simulink model "Lab01R1Sim"  (Simulink 7.1)
settings: Solver=ode45  StartTime=0.0  StopTime=10  RelTol=1e-3
settings Model: Creator=CARLOS BRUNO  LastModifiedBy=CARLOS BRUNO
settings OptimizationCC: InlineInvariantSignals=on
settings DebuggingCC: SaveWithParameterizedLinksMsg=none  SignalResolutionControl=TryResolveAllWithWarning  MultiTaskDSMMsg=warning  MultiTaskCondExecSysMsg=none  StrictBusMsg=None
settings RTWCC: IncludeERTFirstTime=on
settings GRTTargetCC: TargetFcnLib=ansi_tfl_tmw.mat

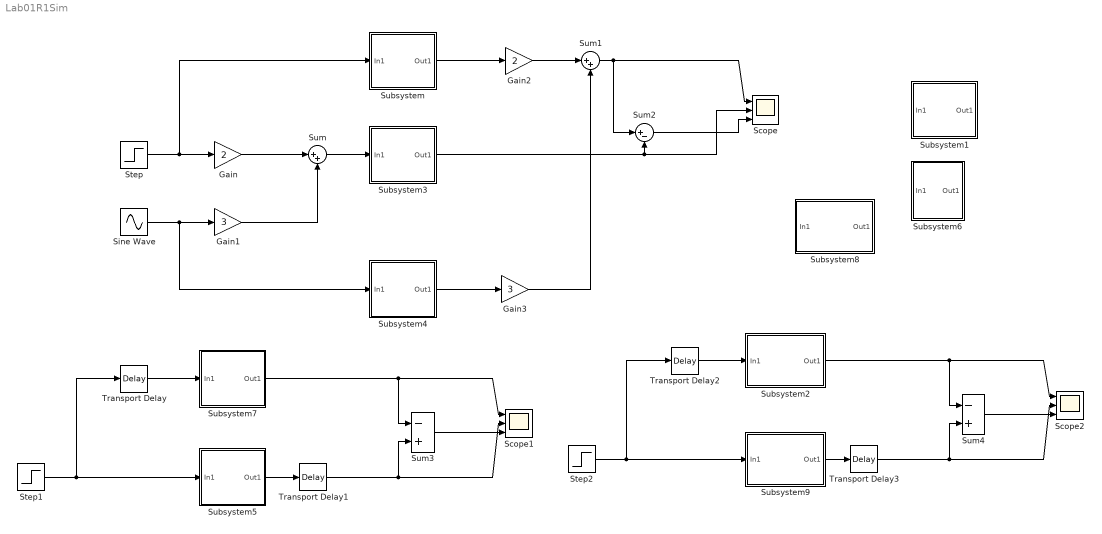
== system Lab01R1Sim ==
  Gain : Gain  Gain=2  ParameterDataType=sfix(16)  ParameterScaling=2^0  OutDataType=sfix(16)  OutScaling=2^0
  Gain1 : Gain  Gain=3  ParameterDataType=sfix(16)  ParameterScaling=2^0  OutDataType=sfix(16)  OutScaling=2^0
  Gain2 : Gain  Gain=2  ParameterDataType=sfix(16)  ParameterScaling=2^0  OutDataType=sfix(16)  OutScaling=2^0
  Gain3 : Gain  Gain=3  ParameterDataType=sfix(16)  ParameterScaling=2^0  OutDataType=sfix(16)  OutScaling=2^0
  Scope : Scope  NumInputPorts=3
      settings: TimeRange=10  YMin=-5~-5~-2e-015  YMax=20~20~4e-015
  Scope1 : Scope  NumInputPorts=3
      settings: TimeRange=10  YMin=-5~-5~-2e-015  YMax=20~20~4e-015
  Scope2 : Scope  NumInputPorts=3
      settings: TimeRange=10  YMin=-5~-5~-2e-015  YMax=20~20~4e-015  SaveName=ScopeData2
  Sine Wave : Sin  SampleTime=0
  Step : Step  Time=0  SampleTime=0
  Step1 : Step  Time=0  SampleTime=0
  Step2 : Step  Time=0  SampleTime=0
  Subsystem : Subsystem
      mask Display: disp('Planta P1')
  Subsystem1 : Subsystem
      mask Display: disp('Planta P2')
  Subsystem2 : Subsystem
      mask Display: disp('Planta P4')
  Subsystem3 : Subsystem
      mask Display: disp('Planta P1')
  Subsystem4 : Subsystem
      mask Display: disp('Planta P1')
  Subsystem5 : Subsystem
      mask Display: disp('Planta P1')
  Subsystem6 : Subsystem
      mask Display: disp('Planta P3')
  Subsystem7 : Subsystem
      mask Display: disp('Planta P1')
  Subsystem8 : Subsystem
      mask Display: disp('Planta P4')
  Subsystem9 : Subsystem
      mask Display: disp('Planta P4')
  Sum : Sum  Inputs=|++  OutDataType=sfix(16)  OutScaling=2^0
  Sum1 : Sum  Inputs=|++  OutDataType=sfix(16)  OutScaling=2^0
  Sum2 : Sum  Inputs=|+-  OutDataType=sfix(16)  OutScaling=2^0
  Sum3 : Sum  Inputs=|-+  OutDataType=sfix(16)  OutScaling=2^0
  Sum4 : Sum  Inputs=|-+  OutDataType=sfix(16)  OutScaling=2^0
  Transport Delay{,1..3} (4 alike) : TransportDelay
  wires:
  Step/1 -> Gain/1, Subsystem/1(In1)
  Sine Wave/1 -> Gain1/1, Subsystem4/1(In1)
  Gain/1 -> Sum/1
  Sum/1 -> Subsystem3/1(In1)
  Gain1/1 -> Sum/2
  Subsystem4/1(Out1) -> Gain3/1
  Subsystem/1(Out1) -> Gain2/1
  Gain2/1 -> Sum1/1
  Gain3/1 -> Sum1/2
  Subsystem3/1(Out1) -> Sum2/2, Scope/2
  Sum1/1 -> Scope/1, Sum2/1
  Sum2/1 -> Scope/3
  Step1/1 -> Transport Delay/1, Subsystem5/1(In1)
  Transport Delay/1 -> Subsystem7/1(In1)
  Subsystem5/1(Out1) -> Transport Delay1/1
  Subsystem7/1(Out1) -> Sum3/1, Scope1/1
  Transport Delay1/1 -> Sum3/2, Scope1/2
  Sum3/1 -> Scope1/3
  Step2/1 -> Transport Delay2/1, Subsystem9/1(In1)
  Transport Delay2/1 -> Subsystem2/1(In1)
  Subsystem2/1(Out1) -> Sum4/1, Scope2/1
  Transport Delay3/1 -> Sum4/2, Scope2/2
  Sum4/1 -> Scope2/3
  Subsystem9/1(Out1) -> Transport Delay3/1

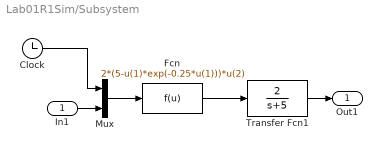
== system Lab01R1Sim/Subsystem ==
  In1 : Inport  OutDataType=sfix(16)  OutScaling=2^0
  Clock : Clock
      settings: Decimation=10
  Fcn : Fcn  Expr=2*(5-u(1)*exp(-0.25*u(1)))*u(2)
  Mux : Mux  Inputs=2
  Transfer Fcn1 : TransferFcn  Numerator=[2]  Denominator=[1 5]
  Out1 : Outport  OutDataType=sfix(16)  OutScaling=2^0
  wires:
  Clock/1 -> Mux/1
  Mux/1 -> Fcn/1
  Fcn/1 -> Transfer Fcn1/1
  Transfer Fcn1/1 -> Out1/1
  In1/1 -> Mux/2

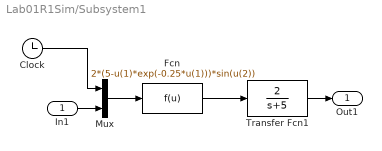
== system Lab01R1Sim/Subsystem1 ==
  In1 : Inport  OutDataType=sfix(16)  OutScaling=2^0
  Clock : Clock
      settings: Decimation=10
  Fcn : Fcn  Expr=2*(5-u(1)*exp(-0.25*u(1)))*sin(u(2))
  Mux : Mux  Inputs=2
  Transfer Fcn1 : TransferFcn  Numerator=[2]  Denominator=[1 5]
  Out1 : Outport  OutDataType=sfix(16)  OutScaling=2^0
  wires:
  Clock/1 -> Mux/1
  Mux/1 -> Fcn/1
  Fcn/1 -> Transfer Fcn1/1
  Transfer Fcn1/1 -> Out1/1
  In1/1 -> Mux/2

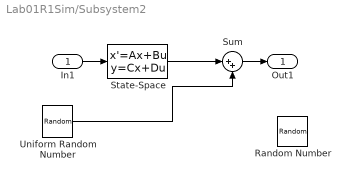
== system Lab01R1Sim/Subsystem2 ==
  In1 : Inport  OutDataType=sfix(16)  OutScaling=2^0
  Random Number : RandomNumber  Variance=0.25  SampleTime=0
  State-Space : StateSpace  A=[-1 -2;1 0]  B=[1; 0]  C="[0  2]"  D=0
  Sum : Sum  Inputs=|++  OutDataType=sfix(16)  OutScaling=2^0
  Uniform Random Number : UniformRandomNumber  Minimum=-0.25  Maximum=0.25  SampleTime=0
  Out1 : Outport  OutDataType=sfix(16)  OutScaling=2^0
  wires:
  State-Space/1 -> Sum/1
  In1/1 -> State-Space/1
  Sum/1 -> Out1/1
  Uniform Random Number/1 -> Sum/2

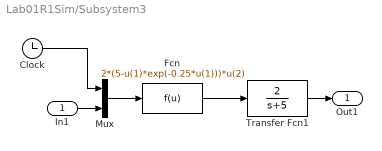
== system Lab01R1Sim/Subsystem3 ==
  In1 : Inport  OutDataType=sfix(16)  OutScaling=2^0
  Clock : Clock
      settings: Decimation=10
  Fcn : Fcn  Expr=2*(5-u(1)*exp(-0.25*u(1)))*u(2)
  Mux : Mux  Inputs=2
  Transfer Fcn1 : TransferFcn  Numerator=[2]  Denominator=[1 5]
  Out1 : Outport  OutDataType=sfix(16)  OutScaling=2^0
  wires:
  Clock/1 -> Mux/1
  Mux/1 -> Fcn/1
  Fcn/1 -> Transfer Fcn1/1
  Transfer Fcn1/1 -> Out1/1
  In1/1 -> Mux/2

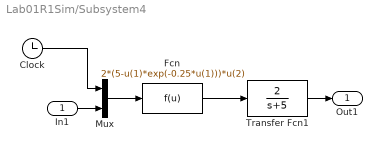
== system Lab01R1Sim/Subsystem4 ==
  In1 : Inport  OutDataType=sfix(16)  OutScaling=2^0
  Clock : Clock
      settings: Decimation=10
  Fcn : Fcn  Expr=2*(5-u(1)*exp(-0.25*u(1)))*u(2)
  Mux : Mux  Inputs=2
  Transfer Fcn1 : TransferFcn  Numerator=[2]  Denominator=[1 5]
  Out1 : Outport  OutDataType=sfix(16)  OutScaling=2^0
  wires:
  Clock/1 -> Mux/1
  Mux/1 -> Fcn/1
  Fcn/1 -> Transfer Fcn1/1
  Transfer Fcn1/1 -> Out1/1
  In1/1 -> Mux/2

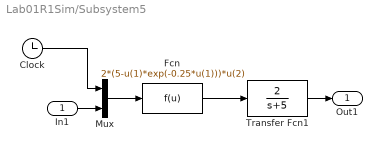
== system Lab01R1Sim/Subsystem5 ==
  In1 : Inport  OutDataType=sfix(16)  OutScaling=2^0
  Clock : Clock
      settings: Decimation=10
  Fcn : Fcn  Expr=2*(5-u(1)*exp(-0.25*u(1)))*u(2)
  Mux : Mux  Inputs=2
  Transfer Fcn1 : TransferFcn  Numerator=[2]  Denominator=[1 5]
  Out1 : Outport  OutDataType=sfix(16)  OutScaling=2^0
  wires:
  Clock/1 -> Mux/1
  Mux/1 -> Fcn/1
  Fcn/1 -> Transfer Fcn1/1
  Transfer Fcn1/1 -> Out1/1
  In1/1 -> Mux/2

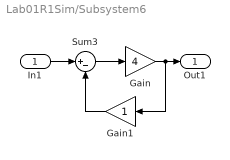
== system Lab01R1Sim/Subsystem6 ==
  In1 : Inport  OutDataType=sfix(16)  OutScaling=2^0
  Gain : Gain  Gain=4  ParameterDataType=sfix(16)  ParameterScaling=2^0  OutDataType=sfix(16)  OutScaling=2^0
  Gain1 : Gain  Orientation=left  ParameterDataType=sfix(16)  ParameterScaling=2^0  OutDataType=sfix(16)  OutScaling=2^0
  Sum3 : Sum  Inputs=|+-  OutDataType=sfix(16)  OutScaling=2^0
  Out1 : Outport  OutDataType=sfix(16)  OutScaling=2^0
  wires:
  Sum3/1 -> Gain/1
  Gain1/1 -> Sum3/2
  Gain/1 -> Out1/1, Gain1/1
  In1/1 -> Sum3/1

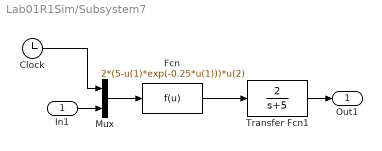
== system Lab01R1Sim/Subsystem7 ==
  In1 : Inport  OutDataType=sfix(16)  OutScaling=2^0
  Clock : Clock
      settings: Decimation=10
  Fcn : Fcn  Expr=2*(5-u(1)*exp(-0.25*u(1)))*u(2)
  Mux : Mux  Inputs=2
  Transfer Fcn1 : TransferFcn  Numerator=[2]  Denominator=[1 5]
  Out1 : Outport  OutDataType=sfix(16)  OutScaling=2^0
  wires:
  Clock/1 -> Mux/1
  Mux/1 -> Fcn/1
  Fcn/1 -> Transfer Fcn1/1
  Transfer Fcn1/1 -> Out1/1
  In1/1 -> Mux/2

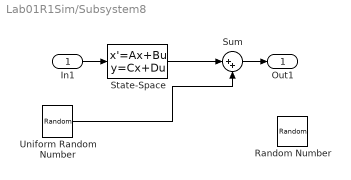
== system Lab01R1Sim/Subsystem8 ==
  In1 : Inport  OutDataType=sfix(16)  OutScaling=2^0
  Random Number : RandomNumber  Variance=0.25  SampleTime=0
  State-Space : StateSpace  A=[-1 -2;1 0]  B=[1; 0]  C="[0  2]"  D=0
  Sum : Sum  Inputs=|++  OutDataType=sfix(16)  OutScaling=2^0
  Uniform Random Number : UniformRandomNumber  Minimum=-0.25  Maximum=0.25  SampleTime=0
  Out1 : Outport  OutDataType=sfix(16)  OutScaling=2^0
  wires:
  State-Space/1 -> Sum/1
  In1/1 -> State-Space/1
  Sum/1 -> Out1/1
  Uniform Random Number/1 -> Sum/2

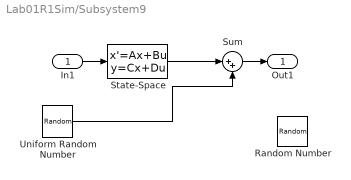
== system Lab01R1Sim/Subsystem9 ==
  In1 : Inport  OutDataType=sfix(16)  OutScaling=2^0
  Random Number : RandomNumber  Variance=0.25  SampleTime=0
  State-Space : StateSpace  A=[-1 -2;1 0]  B=[1; 0]  C="[0  2]"  D=0
  Sum : Sum  Inputs=|++  OutDataType=sfix(16)  OutScaling=2^0
  Uniform Random Number : UniformRandomNumber  Minimum=-0.25  Maximum=0.25  SampleTime=0
  Out1 : Outport  OutDataType=sfix(16)  OutScaling=2^0
  wires:
  State-Space/1 -> Sum/1
  In1/1 -> State-Space/1
  Sum/1 -> Out1/1
  Uniform Random Number/1 -> Sum/2
